simulink model "Auto_Identification_Simulink"  (R2015a)
settings: Solver=ode23t  StartTime=0.0  StopTime=10.0  FixedStep=-0.01  RelTol=1e-3
PostLoadFcn:
  | load('LeftOutput_Measures.mat');
  | load('LeftOutput_Measures.mat');
  | Parametres_Rover
libraries: SingleMotor_Duty_to_inc x2, SingleMotor_V_to_rads x1
settings Model: Creator=tbaroche  LastModifiedBy=tbaroche

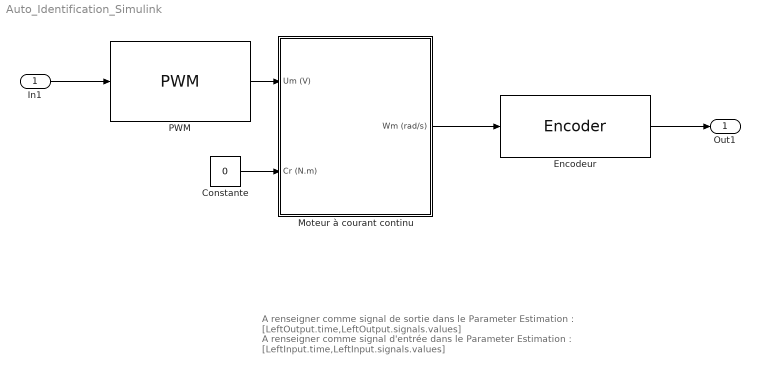
== system Auto_Identification_Simulink ==
  note: A renseigner comme signal d'entrée dans le Parameter Estimation : [LeftInput.time,LeftInput.signals.values]
  note: A renseigner comme signal de sortie dans le Parameter Estimation : [LeftOutput.time,LeftOutput.signals.values]
  In1 : Inport
  Constante : Constant  Value=0
  Encodeur : SingleMotor_Duty_to_inc/Encoder  EncRes=EncRes
  Moteur à courant continu : Subsystem  BlockChoice=Modèle Simulink
      link override "SimElectronics Model ": Kphi_lib=Kphi  Rm_lib=Rm  Lm_lib=Lm  bm_lib=bm  Jm_lib=Jm
      settings: AttributesFormatString=%<BlockChoice>  TemplateBlock=SingleMotor_V_to_rads/DC Motor  MemberBlocks=Modèle Simscape,Modèle Simulink
  PWM : SingleMotor_Duty_to_inc/PWM  FreqTriangle=FreqPWM
  Out1 : Outport
  wires:
  In1/1 -> PWM/1
  Encodeur/1 -> Out1/1
  PWM/1 -> Moteur à courant continu/1(Um (V))
  Moteur à courant continu/1(Wm (rad/s)) -> Encodeur/1
  Constante/1 -> Moteur à courant continu/2(Cr (N.m))

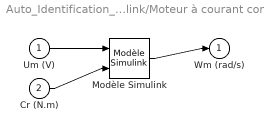
== system Auto_Identification_Simulink/Moteur à courant continu ==
  Um (V) : Inport
  Cr (N.m) : Inport  Port=2
  Modèle Simulink : SingleMotor_V_to_rads/Modèle Simulink  Kphi_lib=Kphi  Rm_lib=Rm  Lm_lib=Lm  bm_lib=bm  Jm_lib=Jm
  Wm (rad/s) : Outport
  wires:
  Um (V)/1 -> Modèle Simulink/1
  Cr (N.m)/1 -> Modèle Simulink/2
  Modèle Simulink/1 -> Wm (rad/s)/1
